simulink model "Es2_sim"  (R2018b)
settings: Solver=VariableStepAuto  StartTime=0.0  StopTime=10.0  RelTol=1e-3
settings Model: Creator=utente  LastModifiedBy=utente

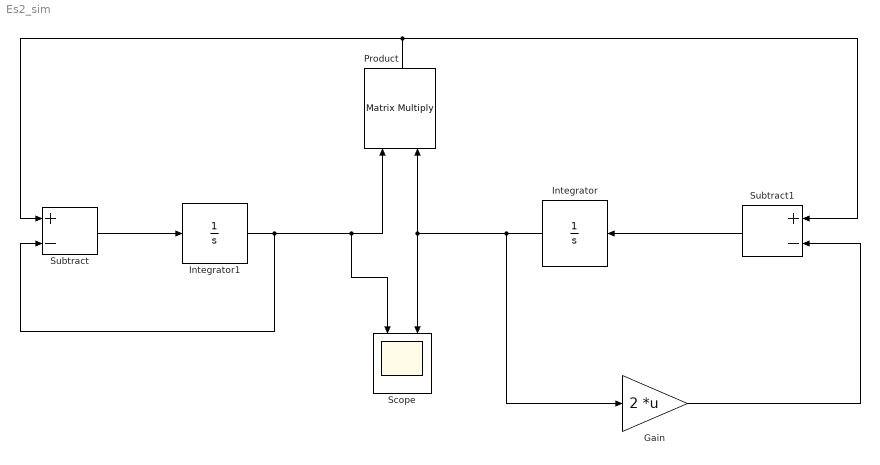
== system Es2_sim ==
  Gain : Gain  Gain=2  Multiplication=Matrix(K*u)
  Integrator : Integrator  InitialCondition=-30
  Integrator1 : Integrator  InitialCondition=-30
  Product : Product  Multiplication=Matrix(*)
  Scope : Scope  NumInputPorts=2
  Subtract : Sum  Inputs=+-
  Subtract1 : Sum  Inputs=+-
  wires:
  Integrator1/1 -> Product/1, Scope/1, Subtract/2
  Integrator/1 -> Scope/2, Product/2, Gain/1
  Product/1 -> Subtract/1, Subtract1/1
  Subtract/1 -> Integrator1/1
  Subtract1/1 -> Integrator/1
  Gain/1 -> Subtract1/2
